simulink model "model_min_mine"  (R2018a)
settings: Solver=ode45  StartTime=0.0  StopTime=20  RelTol=1e-3
(part 8 of 10)

== system model_min_mine/5 систем підйому/4/6-періодні/6-ти періодна пр/постійні ==
  Sum1 : Sum  Inputs=|++++++  SaturateOnIntegerOverflow=on
  Sum2 : Sum  Inputs=|+++  SaturateOnIntegerOverflow=on
  Sum3 : Sum  Inputs=|+++  SaturateOnIntegerOverflow=on
  a1 : Constant  Value=0.5
  a2 : Constant  Value=1.5
  "a4 " : Constant  Value=-1.5
  a5 : Constant  Value=-0.5
  t1 : Constant  Value=0.5
  t2 : Constant  Value=3.5
  t3 : Constant  Value=4
  t4 : Constant  Value=3.5
  "t4/ " : Constant  Value=0.5
  t5 : Constant  Value=0.5
  Out1 : Outport
  Out2 : Outport  Port=2
  Out3 : Outport  Port=3
  Out4 : Outport  Port=4
  Out5 : Outport  Port=5
  Out6 : Outport  Port=6
  Out7 : Outport  Port=7
  Out8 : Outport  Port=8
  Out9 : Outport  Port=9
  Out10 : Outport  Port=10
  wires:
  a1/1 -> Out1/1
  "a4 "/1 -> Out3/1
  a5/1 -> Out4/1
  a2/1 -> Out2/1
  t1/1 -> Out5/1, Sum1/1, Sum2/1
  t3/1 -> Sum1/3, Sum2/3
  t2/1 -> Out6/1, Sum1/2, Sum2/2
  t5/1 -> Sum1/5
  t4/1 -> Out7/1, Sum1/4, Sum3/1
  Sum1/1 -> Out9/1
  Sum2/1 -> Out10/1, Sum3/2
  Sum3/1 -> Out8/1
  "t4/ "/1 -> Sum3/3, Sum1/6

== system model_min_mine/5 систем підйому/4/7-періодні/7-ми періодна криволінійна/Subsystem ==
  t1 : Inport
  t : Inport  Port=2
  a1 : Inport  Port=3
  Constant5 : Constant
  Scope2 : Scope
  Sum4 : Sum  Inputs=|+-  SaturateOnIntegerOverflow=on
  Switch1 : Switch  Criteria=u2 ~= 0  RndMeth=Zero  SaturateOnIntegerOverflow=on
  Генераці : Subsystem  TreatAsAtomicUnit=on
  Out1 : Outport
  wires:
  Генераці/1(Out1) -> Switch1/2
  Sum4/1 -> Генераці/Trigger
  Constant5/1 -> Генераці/1(In1)
  t/1 -> Sum4/2
  t1/1 -> Sum4/1
  Switch1/1 -> Out1/1, Scope2/1
  a1/1 -> Switch1/3

== system model_min_mine/5 систем підйому/4/7-періодні/7-ми періодна криволінійна/Subsystem3 ==
  t1 : Inport
  t : Inport  Port=2
  a1 : Inport  Port=3
  Constant5 : Constant
  Scope2 : Scope
  Sum4 : Sum  Inputs=|+-  SaturateOnIntegerOverflow=on
  Switch1 : Switch  Criteria=u2 ~= 0  RndMeth=Zero  SaturateOnIntegerOverflow=on
  Генераці : Subsystem  TreatAsAtomicUnit=on
  Out1 : Outport
  wires:
  Генераці/1(Out1) -> Switch1/2
  Sum4/1 -> Генераці/Trigger
  Constant5/1 -> Генераці/1(In1)
  t/1 -> Sum4/2
  t1/1 -> Sum4/1
  Switch1/1 -> Out1/1, Scope2/1
  a1/1 -> Switch1/1

== system model_min_mine/5 систем підйому/4/7-періодні/7-ми періодна криволінійна/Subsystem6 ==
  Сума t : Inport
  t : Inport  Port=2
  a : Inport  Port=3
  Constant5 : Constant
  Sum4 : Sum  Inputs=|+-  SaturateOnIntegerOverflow=on
  Switch1 : Switch  Criteria=u2 ~= 0  RndMeth=Zero  SaturateOnIntegerOverflow=on
  Генераці : Subsystem  TreatAsAtomicUnit=on
  Out1 : Outport
  wires:
  Генераці/1(Out1) -> Switch1/2
  Sum4/1 -> Генераці/Trigger
  Constant5/1 -> Генераці/1(In1)
  t/1 -> Sum4/2
  Сума t/1 -> Sum4/1
  Switch1/1 -> Out1/1
  a/1 -> Switch1/3

== system model_min_mine/5 систем підйому/4/7-періодні/7-ми періодна криволінійна/Допоміжний ==
  t1 : Inport
  t : Inport  Port=2
  a1 : Inport  Port=3
  Constant5 : Constant
  Scope2 : Scope
  Sum4 : Sum  Inputs=|+-  SaturateOnIntegerOverflow=on
  Switch1 : Switch  Criteria=u2 ~= 0  RndMeth=Zero  SaturateOnIntegerOverflow=on
  Генераці : Subsystem  TreatAsAtomicUnit=on
  Out1 : Outport
  wires:
  Генераці/1(Out1) -> Switch1/2
  Sum4/1 -> Генераці/Trigger
  Constant5/1 -> Генераці/1(In1)
  t/1 -> Sum4/2
  t1/1 -> Sum4/1
  Switch1/1 -> Out1/1, Scope2/1
  a1/1 -> Switch1/1

== system model_min_mine/5 систем підйому/4/7-періодні/7-ми періодна криволінійна/Допоміжний1 ==
  t1 : Inport
  t : Inport  Port=2
  a1 : Inport  Port=3
  Constant5 : Constant
  Scope2 : Scope
  Sum4 : Sum  Inputs=|+-  SaturateOnIntegerOverflow=on
  Switch1 : Switch  Criteria=u2 ~= 0  RndMeth=Zero  SaturateOnIntegerOverflow=on
  Генераці : Subsystem  TreatAsAtomicUnit=on
  Out1 : Outport
  wires:
  Генераці/1(Out1) -> Switch1/2
  Sum4/1 -> Генераці/Trigger
  Constant5/1 -> Генераці/1(In1)
  t/1 -> Sum4/2
  t1/1 -> Sum4/1
  Switch1/1 -> Out1/1, Scope2/1
  a1/1 -> Switch1/3

== system model_min_mine/5 систем підйому/4/7-періодні/7-ми періодна криволінійна/пакет1 ==
  ti : Inport
  t : Inport  Port=2
  a : Inport  Port=3
  2 : Constant  Value=2
  Math Function1 : Math  Operator=reciprocal  SaturateOnIntegerOverflow=on
  Math Function2 : Math  Operator=reciprocal  SaturateOnIntegerOverflow=on
  Math Function3 : Math  Operator=square  SaturateOnIntegerOverflow=on
  Product10 : Product  Inputs=3  SaturateOnIntegerOverflow=on  OutDataTypeStr=Inherit: Same as first input
  Product3 : Product  Inputs=4  SaturateOnIntegerOverflow=on  OutDataTypeStr=Inherit: Same as first input
  Product4 : Product  SaturateOnIntegerOverflow=on  OutDataTypeStr=Inherit: Same as first input
  Scope1 : Scope
  Scope3 : Scope
  Sum1 : Sum  Inputs=|-+  SaturateOnIntegerOverflow=on
  Sum3 : Sum  Inputs=|+-  SaturateOnIntegerOverflow=on
  Out1 : Outport
  Out2 : Outport  Port=2
  wires:
  Product3/1 -> Sum3/2
  Product4/1 -> Sum3/1
  2/1 -> Math Function2/1
  Math Function1/1 -> Product10/1, Product3/2
  a/1 -> Product4/2, Product3/3, Product10/3, Sum1/2
  ti/1 -> Math Function1/1
  Sum3/1 -> Out2/1, Scope1/1
  Math Function2/1 -> Product3/1
  t/1 -> Math Function3/1, Product10/2, Product4/1
  Math Function3/1 -> Product3/4
  Sum1/1 -> Out1/1, Scope3/1
  Product10/1 -> Sum1/1

== system model_min_mine/5 систем підйому/4/7-періодні/7-ми періодна криволінійна/пакет2 ==
  ti : Inport
  t : Inport  Port=2
  a : Inport  Port=3
  2 : Constant  Value=2
  Math Function1 : Math  Operator=reciprocal  SaturateOnIntegerOverflow=on
  Math Function2 : Math  Operator=reciprocal  SaturateOnIntegerOverflow=on
  Math Function3 : Math  Operator=square  SaturateOnIntegerOverflow=on
  Product10 : Product  Inputs=3  SaturateOnIntegerOverflow=on  OutDataTypeStr=Inherit: Same as first input
  Product3 : Product  Inputs=4  SaturateOnIntegerOverflow=on  OutDataTypeStr=Inherit: Same as first input
  Out1 : Outport
  Out2 : Outport  Port=2
  wires:
  2/1 -> Math Function2/1
  Product10/1 -> Out1/1
  Math Function1/1 -> Product10/1, Product3/2
  a/1 -> Product10/3, Product3/3
  ti/1 -> Math Function1/1
  Math Function2/1 -> Product3/1
  t/1 -> Math Function3/1, Product10/2
  Math Function3/1 -> Product3/4
  Product3/1 -> Out2/1

== system model_min_mine/5 систем підйому/4/7-періодні/7-ми періодна криволінійна/постійні ==
  Sum1 : Sum  Inputs=|+++++++  SaturateOnIntegerOverflow=on
  Sum2 : Sum  Inputs=|+++  SaturateOnIntegerOverflow=on
  Sum3 : Sum  Inputs=|+++  SaturateOnIntegerOverflow=on
  Sum4 : Sum  Inputs=|++  SaturateOnIntegerOverflow=on
  a1 : Constant  Value=0.5
  a2 : Constant  Value=1.5
  "a4 " : Constant  Value=-1.5
  a5 : Constant  Value=-0.5
  t1 : Constant  Value=0.5
  "t1/ " : Constant  Value=0.5
  t2 : Constant  Value=3.5
  t3 : Constant  Value=4
  t4 : Constant  Value=3.5
  "t4/ " : Constant  Value=0.5
  t5 : Constant  Value=0.5
  Out1 : Outport
  Out2 : Outport  Port=2
  Out3 : Outport  Port=3
  Out4 : Outport  Port=4
  Out5 : Outport  Port=5
  Out6 : Outport  Port=6
  Out7 : Outport  Port=7
  Out8 : Outport  Port=8
  Out9 : Outport  Port=9
  Out10 : Outport  Port=10
  Out11 : Outport  Port=11
  wires:
  a1/1 -> Out1/1
  "a4 "/1 -> Out3/1
  a5/1 -> Out4/1
  a2/1 -> Out2/1
  t1/1 -> Out5/1, Sum1/1, Sum2/1, Sum4/1
  t3/1 -> Sum1/3, Sum2/3
  t2/1 -> Out6/1, Sum1/2, Sum2/2
  t5/1 -> Sum1/5
  t4/1 -> Out7/1, Sum1/4, Sum3/1
  Sum1/1 -> Out9/1
  Sum2/1 -> Out10/1, Sum3/2
  Sum3/1 -> Out8/1
  "t4/ "/1 -> Sum3/3, Sum1/6
  "t1/ "/1 -> Sum1/7, Sum4/2
  Sum4/1 -> Out11/1

== system model_min_mine/5 систем підйому/4/7-періодні/7-ми періодна пр/Subsystem ==
  t1 : Inport
  t : Inport  Port=2
  a1 : Inport  Port=3
  Constant5 : Constant
  Scope2 : Scope
  Sum4 : Sum  Inputs=|+-  SaturateOnIntegerOverflow=on
  Switch1 : Switch  Criteria=u2 ~= 0  RndMeth=Zero  SaturateOnIntegerOverflow=on
  Генераці : Subsystem  TreatAsAtomicUnit=on
  Out1 : Outport
  wires:
  Генераці/1(Out1) -> Switch1/2
  Sum4/1 -> Генераці/Trigger
  Constant5/1 -> Генераці/1(In1)
  t/1 -> Sum4/2
  t1/1 -> Sum4/1
  Switch1/1 -> Out1/1, Scope2/1
  a1/1 -> Switch1/3

== system model_min_mine/5 систем підйому/4/7-періодні/7-ми періодна пр/Subsystem1 ==
  t1 : Inport
  t : Inport  Port=2
  a1 : Inport  Port=3
  Constant5 : Constant
  Scope2 : Scope
  Sum4 : Sum  Inputs=|+-  SaturateOnIntegerOverflow=on
  Switch1 : Switch  Criteria=u2 ~= 0  RndMeth=Zero  SaturateOnIntegerOverflow=on
  Генераці : Subsystem  TreatAsAtomicUnit=on
  Out1 : Outport
  wires:
  Генераці/1(Out1) -> Switch1/2
  Sum4/1 -> Генераці/Trigger
  Constant5/1 -> Генераці/1(In1)
  t/1 -> Sum4/2
  t1/1 -> Sum4/1
  Switch1/1 -> Out1/1, Scope2/1
  a1/1 -> Switch1/3

== system model_min_mine/5 систем підйому/4/7-періодні/7-ми періодна пр/Subsystem2 ==
  t1 : Inport
  t : Inport  Port=2
  a1 : Inport  Port=3
  Constant5 : Constant
  Scope2 : Scope
  Scope8 : Scope
  Sum4 : Sum  Inputs=|+-  SaturateOnIntegerOverflow=on
  Switch1 : Switch  Criteria=u2 ~= 0  RndMeth=Zero  SaturateOnIntegerOverflow=on
  Генераці : Subsystem  TreatAsAtomicUnit=on
  Out1 : Outport
  wires:
  Генераці/1(Out1) -> Switch1/2
  Sum4/1 -> Генераці/Trigger
  Constant5/1 -> Генераці/1(In1)
  t/1 -> Sum4/2
  t1/1 -> Sum4/1
  Switch1/1 -> Scope2/1, Out1/1, Scope8/1
  a1/1 -> Switch1/1

== system model_min_mine/5 систем підйому/4/7-періодні/7-ми періодна пр/Subsystem3 ==
  t1 : Inport
  t : Inport  Port=2
  a1 : Inport  Port=3
  Constant5 : Constant
  Scope2 : Scope
  Sum4 : Sum  Inputs=|+-  SaturateOnIntegerOverflow=on
  Switch1 : Switch  Criteria=u2 ~= 0  RndMeth=Zero  SaturateOnIntegerOverflow=on
  Генераці : Subsystem  TreatAsAtomicUnit=on
  Out1 : Outport
  wires:
  Генераці/1(Out1) -> Switch1/2
  Sum4/1 -> Генераці/Trigger
  Constant5/1 -> Генераці/1(In1)
  t/1 -> Sum4/2
  t1/1 -> Sum4/1
  Switch1/1 -> Out1/1, Scope2/1
  a1/1 -> Switch1/1

== system model_min_mine/5 систем підйому/4/7-періодні/7-ми періодна пр/Subsystem6 ==
  Сума t : Inport
  t : Inport  Port=2
  a : Inport  Port=3
  Constant5 : Constant
  Sum4 : Sum  Inputs=|+-  SaturateOnIntegerOverflow=on
  Switch1 : Switch  Criteria=u2 ~= 0  RndMeth=Zero  SaturateOnIntegerOverflow=on
  Генераці : Subsystem  TreatAsAtomicUnit=on
  Out1 : Outport
  wires:
  Генераці/1(Out1) -> Switch1/2
  Sum4/1 -> Генераці/Trigger
  Constant5/1 -> Генераці/1(In1)
  t/1 -> Sum4/2
  Сума t/1 -> Sum4/1
  Switch1/1 -> Out1/1
  a/1 -> Switch1/3

== system model_min_mine/5 систем підйому/4/7-періодні/7-ми періодна пр/Допоміжний ==
  t1 : Inport
  t : Inport  Port=2
  a1 : Inport  Port=3
  Constant5 : Constant
  Scope2 : Scope
  Sum4 : Sum  Inputs=|+-  SaturateOnIntegerOverflow=on
  Switch1 : Switch  Criteria=u2 ~= 0  RndMeth=Zero  SaturateOnIntegerOverflow=on
  Генераці : Subsystem  TreatAsAtomicUnit=on
  Out1 : Outport
  wires:
  Генераці/1(Out1) -> Switch1/2
  Sum4/1 -> Генераці/Trigger
  Constant5/1 -> Генераці/1(In1)
  t/1 -> Sum4/2
  t1/1 -> Sum4/1
  Switch1/1 -> Out1/1, Scope2/1
  a1/1 -> Switch1/1

== system model_min_mine/5 систем підйому/4/7-періодні/7-ми періодна пр/Допоміжний1 ==
  t1 : Inport
  t : Inport  Port=2
  a1 : Inport  Port=3
  Constant5 : Constant
  Scope2 : Scope
  Sum4 : Sum  Inputs=|+-  SaturateOnIntegerOverflow=on
  Switch1 : Switch  Criteria=u2 ~= 0  RndMeth=Zero  SaturateOnIntegerOverflow=on
  Генераці : Subsystem  TreatAsAtomicUnit=on
  Out1 : Outport
  wires:
  Генераці/1(Out1) -> Switch1/2
  Sum4/1 -> Генераці/Trigger
  Constant5/1 -> Генераці/1(In1)
  t/1 -> Sum4/2
  t1/1 -> Sum4/1
  Switch1/1 -> Out1/1, Scope2/1
  a1/1 -> Switch1/3

== system model_min_mine/5 систем підйому/4/7-періодні/7-ми періодна пр/постійні ==
  Sum1 : Sum  Inputs=|+++++++  SaturateOnIntegerOverflow=on
  Sum2 : Sum  Inputs=|+++  SaturateOnIntegerOverflow=on
  Sum3 : Sum  Inputs=|+++  SaturateOnIntegerOverflow=on
  Sum4 : Sum  Inputs=|++  SaturateOnIntegerOverflow=on
  a1 : Constant  Value=0.5
  a2 : Constant  Value=1.5
  "a4 " : Constant  Value=-1.5
  a5 : Constant  Value=-0.5
  t1 : Constant  Value=0.5
  "t1/ " : Constant  Value=0.5
  t2 : Constant  Value=3.5
  t3 : Constant  Value=8
  t4 : Constant  Value=3.5
  "t4/ " : Constant  Value=0.5
  t5 : Constant  Value=0.5
  Out1 : Outport
  Out2 : Outport  Port=2
  Out3 : Outport  Port=3
  Out4 : Outport  Port=4
  Out5 : Outport  Port=5
  Out6 : Outport  Port=6
  Out7 : Outport  Port=7
  Out8 : Outport  Port=8
  Out9 : Outport  Port=9
  Out10 : Outport  Port=10
  Out11 : Outport  Port=11
  wires:
  a1/1 -> Out1/1
  "a4 "/1 -> Out3/1
  a5/1 -> Out4/1
  a2/1 -> Out2/1
  t1/1 -> Out5/1, Sum1/1, Sum2/1, Sum4/1
  t3/1 -> Sum1/3, Sum2/3
  t2/1 -> Out6/1, Sum1/2, Sum2/2
  t5/1 -> Sum1/5
  t4/1 -> Out7/1, Sum1/4, Sum3/1
  Sum1/1 -> Out9/1
  Sum2/1 -> Out10/1, Sum3/2
  Sum3/1 -> Out8/1
  "t4/ "/1 -> Sum3/3, Sum1/6
  "t1/ "/1 -> Sum1/7, Sum4/2
  Sum4/1 -> Out11/1

== system model_min_mine/5 систем підйому/6/3-періодні/Криволінійна-3/Генераці1 ==
  In1 : Inport
  Trigger : TriggerPort  TriggerType=either  VariantControl=(inherit)  ShowOutputPort=on
  Out1 : Outport
  wires:
  In1/1 -> Out1/1

== system model_min_mine/5 систем підйому/6/3-періодні/Криволінійна-3/пакет2 ==
  ti : Inport
  t : Inport  Port=2
  a : Inport  Port=3
  2 : Constant  Value=2
  Math Function1 : Math  Operator=reciprocal  SaturateOnIntegerOverflow=on
  Math Function2 : Math  Operator=reciprocal  SaturateOnIntegerOverflow=on
  Math Function3 : Math  Operator=square  SaturateOnIntegerOverflow=on
  Product10 : Product  Inputs=3  SaturateOnIntegerOverflow=on  OutDataTypeStr=Inherit: Same as first input
  Product3 : Product  Inputs=4  SaturateOnIntegerOverflow=on  OutDataTypeStr=Inherit: Same as first input
  Product4 : Product  SaturateOnIntegerOverflow=on  OutDataTypeStr=Inherit: Same as first input
  Scope1 : Scope
  Scope3 : Scope
  Sum1 : Sum  Inputs=|-+  SaturateOnIntegerOverflow=on
  Sum3 : Sum  Inputs=|+-  SaturateOnIntegerOverflow=on
  Out1 : Outport
  Out2 : Outport  Port=2
  wires:
  Product3/1 -> Sum3/2
  Product4/1 -> Sum3/1
  2/1 -> Math Function2/1
  Math Function1/1 -> Product10/1, Product3/2
  a/1 -> Product4/2, Product3/3, Product10/3, Sum1/2
  ti/1 -> Math Function1/1
  Sum3/1 -> Out2/1, Scope1/1
  Math Function2/1 -> Product3/1
  t/1 -> Math Function3/1, Product10/2, Product4/1
  Math Function3/1 -> Product3/4
  Sum1/1 -> Out1/1, Scope3/1
  Product10/1 -> Sum1/1

== system model_min_mine/5 систем підйому/6/3-періодні/Криволінійна-3/пакет3 ==
  ti : Inport
  t : Inport  Port=2
  a : Inport  Port=3
  2 : Constant  Value=2
  Math Function1 : Math  Operator=reciprocal  SaturateOnIntegerOverflow=on
  Math Function2 : Math  Operator=reciprocal  SaturateOnIntegerOverflow=on
  Math Function3 : Math  Operator=square  SaturateOnIntegerOverflow=on
  Product10 : Product  Inputs=3  SaturateOnIntegerOverflow=on  OutDataTypeStr=Inherit: Same as first input
  Product3 : Product  Inputs=4  SaturateOnIntegerOverflow=on  OutDataTypeStr=Inherit: Same as first input
  Out1 : Outport
  Out2 : Outport  Port=2
  wires:
  2/1 -> Math Function2/1
  Product10/1 -> Out1/1
  Math Function1/1 -> Product10/1, Product3/2
  a/1 -> Product10/3, Product3/3
  ti/1 -> Math Function1/1
  Math Function2/1 -> Product3/1
  t/1 -> Math Function3/1, Product10/2
  Math Function3/1 -> Product3/4
  Product3/1 -> Out2/1

== system model_min_mine/5 систем підйому/6/3-періодні/Криволінійна-3/постійні ==
  a1 : Constant  Value=0.3
  a3 : Constant  Value=-0.3
  t1 : Constant  Value=1.15
  t3 : Constant  Value=1.15
  Out1 : Outport
  Out2 : Outport  Port=2
  Out3 : Outport  Port=3
  Out4 : Outport  Port=4
  wires:
  a1/1 -> Out1/1
  t1/1 -> Out3/1
  a3/1 -> Out2/1
  t3/1 -> Out4/1

== system model_min_mine/5 систем підйому/6/3-періодні/Пр/Генераці ==
  In1 : Inport
  Trigger : TriggerPort  TriggerType=either  VariantControl=(inherit)  ShowOutputPort=on
  Out1 : Outport
  wires:
  In1/1 -> Out1/1

== system model_min_mine/5 систем підйому/6/3-періодні/Пр/Генераці1 ==
  In1 : Inport
  Trigger : TriggerPort  TriggerType=either  VariantControl=(inherit)  ShowOutputPort=on
  Out1 : Outport
  wires:
  In1/1 -> Out1/1

== system model_min_mine/5 систем підйому/6/3-періодні/Пр/Генераці2 ==
  In1 : Inport
  Trigger : TriggerPort  TriggerType=either  VariantControl=(inherit)  ShowOutputPort=on
  Out1 : Outport
  wires:
  In1/1 -> Out1/1

== system model_min_mine/5 систем підйому/6/3-періодні/Пр/постійні ==
  (t1) : Constant  Value=1.15
  (t2) : Constant  Value=2
  (t3) : Constant  Value=1.15
  Sum1 : Sum  Inputs=|++  SaturateOnIntegerOverflow=on
  a1 : Constant  Value=0.3
  a3 : Constant  Value=-0.3
  Out1 : Outport
  Out2 : Outport  Port=2
  Out3 : Outport  Port=3
  Out4 : Outport  Port=4
  Out5 : Outport  Port=5
  wires:
  a1/1 -> Out1/1
  a3/1 -> Out2/1
  (t3)/1 -> Out3/1
  (t1)/1 -> Out4/1, Sum1/1
  (t2)/1 -> Sum1/2
  Sum1/1 -> Out5/1

== system model_min_mine/5 систем підйому/6/5-періодні/криво/Subsystem ==
  t1 : Inport
  t : Inport  Port=2
  a1 : Inport  Port=3
  Constant5 : Constant
  Scope2 : Scope
  Sum4 : Sum  Inputs=|+-  SaturateOnIntegerOverflow=on
  Switch1 : Switch  Criteria=u2 ~= 0  RndMeth=Zero  SaturateOnIntegerOverflow=on
  Генераці : Subsystem  TreatAsAtomicUnit=on
  Out1 : Outport
  wires:
  Генераці/1(Out1) -> Switch1/2
  Sum4/1 -> Генераці/Trigger
  Constant5/1 -> Генераці/1(In1)
  t/1 -> Sum4/2
  t1/1 -> Sum4/1
  Switch1/1 -> Out1/1, Scope2/1
  a1/1 -> Switch1/3

== system model_min_mine/5 систем підйому/6/5-періодні/криво/Subsystem1 ==
  t1 : Inport
  t : Inport  Port=2
  a1 : Inport  Port=3
  Constant5 : Constant
  Scope2 : Scope
  Sum4 : Sum  Inputs=|+-  SaturateOnIntegerOverflow=on
  Switch1 : Switch  Criteria=u2 ~= 0  RndMeth=Zero  SaturateOnIntegerOverflow=on
  Генераці : Subsystem  TreatAsAtomicUnit=on
  Out1 : Outport
  wires:
  Генераці/1(Out1) -> Switch1/2
  Sum4/1 -> Генераці/Trigger
  Constant5/1 -> Генераці/1(In1)
  t/1 -> Sum4/2
  t1/1 -> Sum4/1
  Switch1/1 -> Out1/1, Scope2/1
  a1/1 -> Switch1/3

== system model_min_mine/5 систем підйому/6/5-періодні/криво/Subsystem2 ==
  t1 : Inport
  t : Inport  Port=2
  a1 : Inport  Port=3
  Constant5 : Constant
  Scope2 : Scope
  Scope8 : Scope
  Sum4 : Sum  Inputs=|+-  SaturateOnIntegerOverflow=on
  Switch1 : Switch  Criteria=u2 ~= 0  RndMeth=Zero  SaturateOnIntegerOverflow=on
  Генераці : Subsystem  TreatAsAtomicUnit=on
  Out1 : Outport
  wires:
  Генераці/1(Out1) -> Switch1/2
  Sum4/1 -> Генераці/Trigger
  Constant5/1 -> Генераці/1(In1)
  t/1 -> Sum4/2
  t1/1 -> Sum4/1
  Switch1/1 -> Scope2/1, Out1/1, Scope8/1
  a1/1 -> Switch1/1

== system model_min_mine/5 систем підйому/6/5-періодні/криво/Subsystem3 ==
  t1 : Inport
  t : Inport  Port=2
  a1 : Inport  Port=3
  Constant5 : Constant
  Scope2 : Scope
  Sum4 : Sum  Inputs=|+-  SaturateOnIntegerOverflow=on
  Switch1 : Switch  Criteria=u2 ~= 0  RndMeth=Zero  SaturateOnIntegerOverflow=on
  Генераці : Subsystem  TreatAsAtomicUnit=on
  Out1 : Outport
  wires:
  Генераці/1(Out1) -> Switch1/2
  Sum4/1 -> Генераці/Trigger
  Constant5/1 -> Генераці/1(In1)
  t/1 -> Sum4/2
  t1/1 -> Sum4/1
  Switch1/1 -> Out1/1, Scope2/1
  a1/1 -> Switch1/1

== system model_min_mine/5 систем підйому/6/5-періодні/криво/Subsystem6 ==
  Сума t : Inport
  t : Inport  Port=2
  a : Inport  Port=3
  Constant5 : Constant
  Sum4 : Sum  Inputs=|+-  SaturateOnIntegerOverflow=on
  Switch1 : Switch  Criteria=u2 ~= 0  RndMeth=Zero  SaturateOnIntegerOverflow=on
  Генераці : Subsystem  TreatAsAtomicUnit=on
  Out1 : Outport
  wires:
  Генераці/1(Out1) -> Switch1/2
  Sum4/1 -> Генераці/Trigger
  Constant5/1 -> Генераці/1(In1)
  t/1 -> Sum4/2
  Сума t/1 -> Sum4/1
  Switch1/1 -> Out1/1
  a/1 -> Switch1/3

== system model_min_mine/5 систем підйому/6/5-періодні/криво/Допоміжний ==
  t1 : Inport
  t : Inport  Port=2
  a1 : Inport  Port=3
  Constant5 : Constant
  Scope2 : Scope
  Sum4 : Sum  Inputs=|+-  SaturateOnIntegerOverflow=on
  Switch1 : Switch  Criteria=u2 ~= 0  RndMeth=Zero  SaturateOnIntegerOverflow=on
  Генераці : Subsystem  TreatAsAtomicUnit=on
  Out1 : Outport
  wires:
  Генераці/1(Out1) -> Switch1/2
  Sum4/1 -> Генераці/Trigger
  Constant5/1 -> Генераці/1(In1)
  t/1 -> Sum4/2
  t1/1 -> Sum4/1
  Switch1/1 -> Out1/1, Scope2/1
  a1/1 -> Switch1/1

== system model_min_mine/5 систем підйому/6/5-періодні/криво/Допоміжний1 ==
  t1 : Inport
  t : Inport  Port=2
  a1 : Inport  Port=3
  Constant5 : Constant
  Scope2 : Scope
  Sum4 : Sum  Inputs=|+-  SaturateOnIntegerOverflow=on
  Switch1 : Switch  Criteria=u2 ~= 0  RndMeth=Zero  SaturateOnIntegerOverflow=on
  Генераці : Subsystem  TreatAsAtomicUnit=on
  Out1 : Outport
  wires:
  Генераці/1(Out1) -> Switch1/2
  Sum4/1 -> Генераці/Trigger
  Constant5/1 -> Генераці/1(In1)
  t/1 -> Sum4/2
  t1/1 -> Sum4/1
  Switch1/1 -> Out1/1, Scope2/1
  a1/1 -> Switch1/3

== system model_min_mine/5 систем підйому/6/5-періодні/криво/постійні ==
  Sum1 : Sum  Inputs=|+++++  SaturateOnIntegerOverflow=on
  Sum2 : Sum  Inputs=|+++  SaturateOnIntegerOverflow=on
  Sum3 : Sum  Inputs=|++  SaturateOnIntegerOverflow=on
  a1 : Constant  Value=0.5
  a2 : Constant  Value=1.5
  "a4 " : Constant  Value=-1.5
  a5 : Constant  Value=-0.5
  t1 : Constant  Value=0.5
  t2 : Constant  Value=3.5
  t3 : Constant  Value=4
  t4 : Constant  Value=3.5
  t5 : Constant  Value=0.5
  Out1 : Outport
  Out2 : Outport  Port=2
  Out3 : Outport  Port=3
  Out4 : Outport  Port=4
  Out5 : Outport  Port=5
  Out6 : Outport  Port=6
  Out7 : Outport  Port=7
  Out8 : Outport  Port=8
  Out9 : Outport  Port=9
  Out10 : Outport  Port=10
  wires:
  a1/1 -> Out1/1
  "a4 "/1 -> Out3/1
  a5/1 -> Out4/1
  a2/1 -> Out2/1
  t1/1 -> Out5/1, Sum1/1, Sum2/1
  t3/1 -> Sum1/3, Sum2/3
  t2/1 -> Out6/1, Sum1/2, Sum2/2
  t5/1 -> Sum1/5
  t4/1 -> Out7/1, Sum1/4, Sum3/1
  Sum1/1 -> Out9/1
  Sum2/1 -> Out10/1, Sum3/2
  Sum3/1 -> Out8/1

== system model_min_mine/5 систем підйому/6/5-періодні/пр/Subsystem ==
  t1 : Inport
  t : Inport  Port=2
  a1 : Inport  Port=3
  Constant5 : Constant
  Scope2 : Scope
  Sum4 : Sum  Inputs=|+-  SaturateOnIntegerOverflow=on
  Switch1 : Switch  Criteria=u2 ~= 0  RndMeth=Zero  SaturateOnIntegerOverflow=on
  Генераці : Subsystem  TreatAsAtomicUnit=on
  Out1 : Outport
  wires:
  Генераці/1(Out1) -> Switch1/2
  Sum4/1 -> Генераці/Trigger
  Constant5/1 -> Генераці/1(In1)
  t/1 -> Sum4/2
  t1/1 -> Sum4/1
  Switch1/1 -> Out1/1, Scope2/1
  a1/1 -> Switch1/3

== system model_min_mine/5 систем підйому/6/5-періодні/пр/Subsystem1 ==
  t1 : Inport
  t : Inport  Port=2
  a1 : Inport  Port=3
  Constant5 : Constant
  Scope2 : Scope
  Sum4 : Sum  Inputs=|+-  SaturateOnIntegerOverflow=on
  Switch1 : Switch  Criteria=u2 ~= 0  RndMeth=Zero  SaturateOnIntegerOverflow=on
  Генераці : Subsystem  TreatAsAtomicUnit=on
  Out1 : Outport
  wires:
  Генераці/1(Out1) -> Switch1/2
  Sum4/1 -> Генераці/Trigger
  Constant5/1 -> Генераці/1(In1)
  t/1 -> Sum4/2
  t1/1 -> Sum4/1
  Switch1/1 -> Out1/1, Scope2/1
  a1/1 -> Switch1/3

== system model_min_mine/5 систем підйому/6/5-періодні/пр/Subsystem4 ==
  ti : Inport
  t : Inport  Port=2
  a : Inport  Port=3
  Constant5 : Constant
  Sum4 : Sum  Inputs=|+-  SaturateOnIntegerOverflow=on
  Switch1 : Switch  Criteria=u2 ~= 0  RndMeth=Zero  SaturateOnIntegerOverflow=on
  Генераці : Subsystem  TreatAsAtomicUnit=on
  Out1 : Outport
  wires:
  Генераці/1(Out1) -> Switch1/2
  Sum4/1 -> Генераці/Trigger
  Constant5/1 -> Генераці/1(In1)
  t/1 -> Sum4/2
  ti/1 -> Sum4/1
  a/1 -> Switch1/1
  Switch1/1 -> Out1/1

== system model_min_mine/5 систем підйому/6/5-періодні/пр/Subsystem5 ==
  ti : Inport
  t : Inport  Port=2
  a : Inport  Port=3
  Constant5 : Constant
  Sum4 : Sum  Inputs=|+-  SaturateOnIntegerOverflow=on
  Switch1 : Switch  Criteria=u2 ~= 0  RndMeth=Zero  SaturateOnIntegerOverflow=on
  Генераці : Subsystem  TreatAsAtomicUnit=on
  Out1 : Outport
  wires:
  Генераці/1(Out1) -> Switch1/2
  Sum4/1 -> Генераці/Trigger
  Constant5/1 -> Генераці/1(In1)
  t/1 -> Sum4/2
  ti/1 -> Sum4/1
  a/1 -> Switch1/1
  Switch1/1 -> Out1/1

== system model_min_mine/5 систем підйому/6/5-періодні/пр/Subsystem6 ==
  Сума t : Inport
  t : Inport  Port=2
  a : Inport  Port=3
  Constant5 : Constant
  Sum4 : Sum  Inputs=|+-  SaturateOnIntegerOverflow=on
  Switch1 : Switch  Criteria=u2 ~= 0  RndMeth=Zero  SaturateOnIntegerOverflow=on
  Генераці : Subsystem  TreatAsAtomicUnit=on
  Out1 : Outport
  wires:
  Генераці/1(Out1) -> Switch1/2
  Sum4/1 -> Генераці/Trigger
  Constant5/1 -> Генераці/1(In1)
  t/1 -> Sum4/2
  Сума t/1 -> Sum4/1
  Switch1/1 -> Out1/1
  a/1 -> Switch1/3

== system model_min_mine/5 систем підйому/6/5-періодні/пр/Допоміжний ==
  t1 : Inport
  t : Inport  Port=2
  a1 : Inport  Port=3
  Constant5 : Constant
  Scope2 : Scope
  Sum4 : Sum  Inputs=|+-  SaturateOnIntegerOverflow=on
  Switch1 : Switch  Criteria=u2 ~= 0  RndMeth=Zero  SaturateOnIntegerOverflow=on
  Генераці : Subsystem  TreatAsAtomicUnit=on
  Out1 : Outport
  wires:
  Генераці/1(Out1) -> Switch1/2
  Sum4/1 -> Генераці/Trigger
  Constant5/1 -> Генераці/1(In1)
  t/1 -> Sum4/2
  t1/1 -> Sum4/1
  Switch1/1 -> Out1/1, Scope2/1
  a1/1 -> Switch1/1

== system model_min_mine/5 систем підйому/6/5-періодні/пр/Допоміжний -1 ==
  t1 : Inport
  t : Inport  Port=2
  a1 : Inport  Port=3
  Constant5 : Constant
  Scope2 : Scope
  Sum4 : Sum  Inputs=|+-  SaturateOnIntegerOverflow=on
  Switch1 : Switch  Criteria=u2 ~= 0  RndMeth=Zero  SaturateOnIntegerOverflow=on
  Генераці : Subsystem  TreatAsAtomicUnit=on
  Out1 : Outport
  wires:
  Генераці/1(Out1) -> Switch1/2
  Sum4/1 -> Генераці/Trigger
  Constant5/1 -> Генераці/1(In1)
  t/1 -> Sum4/2
  t1/1 -> Sum4/1
  Switch1/1 -> Out1/1, Scope2/1
  a1/1 -> Switch1/1

== system model_min_mine/5 систем підйому/6/5-періодні/пр/Допоміжний -2 ==
  t1 : Inport
  t : Inport  Port=2
  a1 : Inport  Port=3
  Constant5 : Constant
  Scope2 : Scope
  Sum4 : Sum  Inputs=|+-  SaturateOnIntegerOverflow=on
  Switch1 : Switch  Criteria=u2 ~= 0  RndMeth=Zero  SaturateOnIntegerOverflow=on
  Генераці : Subsystem  TreatAsAtomicUnit=on
  Out1 : Outport
  wires:
  Генераці/1(Out1) -> Switch1/2
  Sum4/1 -> Генераці/Trigger
  Constant5/1 -> Генераці/1(In1)
  t/1 -> Sum4/2
  t1/1 -> Sum4/1
  Switch1/1 -> Out1/1, Scope2/1
  a1/1 -> Switch1/1

== system model_min_mine/5 систем підйому/6/5-періодні/пр/Допоміжний -3 ==
  t1 : Inport
  t : Inport  Port=2
  a1 : Inport  Port=3
  Constant5 : Constant
  Scope2 : Scope
  Sum4 : Sum  Inputs=|+-  SaturateOnIntegerOverflow=on
  Switch1 : Switch  Criteria=u2 ~= 0  RndMeth=Zero  SaturateOnIntegerOverflow=on
  Генераці : Subsystem  TreatAsAtomicUnit=on
  Out1 : Outport
  wires:
  Генераці/1(Out1) -> Switch1/2
  Sum4/1 -> Генераці/Trigger
  Constant5/1 -> Генераці/1(In1)
  t/1 -> Sum4/2
  t1/1 -> Sum4/1
  Switch1/1 -> Out1/1, Scope2/1
  a1/1 -> Switch1/1

== system model_min_mine/5 систем підйому/6/5-періодні/пр/Допоміжний -4 ==
  t1 : Inport
  t : Inport  Port=2
  a1 : Inport  Port=3
  Constant5 : Constant
  Scope2 : Scope
  Sum4 : Sum  Inputs=|+-  SaturateOnIntegerOverflow=on
  Switch1 : Switch  Criteria=u2 ~= 0  RndMeth=Zero  SaturateOnIntegerOverflow=on
  Генераці : Subsystem  TreatAsAtomicUnit=on
  Out1 : Outport
  wires:
  Генераці/1(Out1) -> Switch1/2
  Sum4/1 -> Генераці/Trigger
  Constant5/1 -> Генераці/1(In1)
  t/1 -> Sum4/2
  t1/1 -> Sum4/1
  Switch1/1 -> Out1/1, Scope2/1
  a1/1 -> Switch1/1

== system model_min_mine/5 систем підйому/6/5-періодні/пр/пакет1 ==
  ti : Inport
  t : Inport  Port=2
  a : Inport  Port=3
  2 : Constant  Value=2
  Math Function1 : Math  Operator=reciprocal  SaturateOnIntegerOverflow=on
  Math Function2 : Math  Operator=reciprocal  SaturateOnIntegerOverflow=on
  Math Function3 : Math  Operator=square  SaturateOnIntegerOverflow=on
  Product10 : Product  Inputs=3  SaturateOnIntegerOverflow=on  OutDataTypeStr=Inherit: Same as first input
  Product3 : Product  Inputs=4  SaturateOnIntegerOverflow=on  OutDataTypeStr=Inherit: Same as first input
  Product4 : Product  SaturateOnIntegerOverflow=on  OutDataTypeStr=Inherit: Same as first input
  Scope3 : Scope
  Sum1 : Sum  Inputs=|-+  SaturateOnIntegerOverflow=on
  Sum3 : Sum  Inputs=|+-  SaturateOnIntegerOverflow=on
  Out1 : Outport
  Out2 : Outport  Port=2
  wires:
  Product3/1 -> Sum3/2
  Product4/1 -> Sum3/1
  2/1 -> Math Function2/1
  Math Function1/1 -> Product10/1, Product3/2
  a/1 -> Product4/2, Product3/3, Product10/3, Sum1/2
  ti/1 -> Math Function1/1
  Sum3/1 -> Out2/1
  Math Function2/1 -> Product3/1
  t/1 -> Math Function3/1, Product10/2, Product4/1
  Math Function3/1 -> Product3/4
  Sum1/1 -> Out1/1, Scope3/1
  Product10/1 -> Sum1/1

== system model_min_mine/5 систем підйому/6/5-періодні/пр/пакет2 ==
  ti : Inport
  t : Inport  Port=2
  a : Inport  Port=3
  2 : Constant  Value=2
  Math Function1 : Math  Operator=reciprocal  SaturateOnIntegerOverflow=on
  Math Function2 : Math  Operator=reciprocal  SaturateOnIntegerOverflow=on
  Math Function3 : Math  Operator=square  SaturateOnIntegerOverflow=on
  Product10 : Product  Inputs=3  SaturateOnIntegerOverflow=on  OutDataTypeStr=Inherit: Same as first input
  Product3 : Product  Inputs=4  SaturateOnIntegerOverflow=on  OutDataTypeStr=Inherit: Same as first input
  Out1 : Outport
  Out2 : Outport  Port=2
  wires:
  2/1 -> Math Function2/1
  Product10/1 -> Out1/1
  Math Function1/1 -> Product10/1, Product3/2
  a/1 -> Product10/3, Product3/3
  ti/1 -> Math Function1/1
  Math Function2/1 -> Product3/1
  t/1 -> Math Function3/1, Product10/2
  Math Function3/1 -> Product3/4
  Product3/1 -> Out2/1

== system model_min_mine/5 систем підйому/6/5-періодні/пр/постійні ==
  Sum1 : Sum  Inputs=|+++++++  SaturateOnIntegerOverflow=on
  a1 : Constant  Value=0.5
  a2 : Constant  Value=1.5
  "a3 " : Constant  Value=1.5
  a5 на кінці : Constant  Value=-1.5
  a6 : Constant  Value=-1.5
  a7 : Constant  Value=-0.5
  t{1,3,5,7} (4 alike) : Constant  Value=0.5
  t2 : Constant  Value=3.5
  t4 : Constant  Value=3
  t6 : Constant  Value=3.5
  Out1 : Outport
  Out2 : Outport  Port=2
  Out3 : Outport  Port=3
  Out4 : Outport  Port=4
  Out5 : Outport  Port=5
  Out6 : Outport  Port=6
  Out7 : Outport  Port=7
  Out8 : Outport  Port=8
  Out9 : Outport  Port=9
  Out10 : Outport  Port=10
  Out11 : Outport  Port=11
  Out12 : Outport  Port=12
  Out13 : Outport  Port=13
  wires:
  a1/1 -> Out1/1
  "a3 "/1 -> Out3/1
  a5 на кінці/1 -> Out4/1
  a2/1 -> Out2/1
  a6/1 -> Out5/1
  a7/1 -> Out6/1
  t1/1 -> Out7/1, Sum1/1
  t3/1 -> Out9/1, Sum1/3
  t2/1 -> Out8/1, Sum1/2
  t5/1 -> Out11/1, Sum1/5
  t6/1 -> Out12/1, Sum1/6
  t7/1 -> Out13/1, Sum1/7
  t4/1 -> Sum1/4
  Sum1/1 -> Out10/1

== system model_min_mine/5 систем підйому/6/6-періодні/6-ти періодна криволінійна/Subsystem ==
  t1 : Inport
  t : Inport  Port=2
  a1 : Inport  Port=3
  Constant5 : Constant
  Scope2 : Scope
  Sum4 : Sum  Inputs=|+-  SaturateOnIntegerOverflow=on
  Switch1 : Switch  Criteria=u2 ~= 0  RndMeth=Zero  SaturateOnIntegerOverflow=on
  Генераці : Subsystem  TreatAsAtomicUnit=on
  Out1 : Outport
  wires:
  Генераці/1(Out1) -> Switch1/2
  Sum4/1 -> Генераці/Trigger
  Constant5/1 -> Генераці/1(In1)
  t/1 -> Sum4/2
  t1/1 -> Sum4/1
  Switch1/1 -> Out1/1, Scope2/1
  a1/1 -> Switch1/3

== system model_min_mine/5 систем підйому/6/6-періодні/6-ти періодна криволінійна/Subsystem3 ==
  t1 : Inport
  t : Inport  Port=2
  a1 : Inport  Port=3
  Constant5 : Constant
  Scope2 : Scope
  Sum4 : Sum  Inputs=|+-  SaturateOnIntegerOverflow=on
  Switch1 : Switch  Criteria=u2 ~= 0  RndMeth=Zero  SaturateOnIntegerOverflow=on
  Генераці : Subsystem  TreatAsAtomicUnit=on
  Out1 : Outport
  wires:
  Генераці/1(Out1) -> Switch1/2
  Sum4/1 -> Генераці/Trigger
  Constant5/1 -> Генераці/1(In1)
  t/1 -> Sum4/2
  t1/1 -> Sum4/1
  Switch1/1 -> Out1/1, Scope2/1
  a1/1 -> Switch1/1

== system model_min_mine/5 систем підйому/6/6-періодні/6-ти періодна криволінійна/Subsystem6 ==
  Сума t : Inport
  t : Inport  Port=2
  a : Inport  Port=3
  Constant5 : Constant
  Sum4 : Sum  Inputs=|+-  SaturateOnIntegerOverflow=on
  Switch1 : Switch  Criteria=u2 ~= 0  RndMeth=Zero  SaturateOnIntegerOverflow=on
  Генераці : Subsystem  TreatAsAtomicUnit=on
  Out1 : Outport
  wires:
  Генераці/1(Out1) -> Switch1/2
  Sum4/1 -> Генераці/Trigger
  Constant5/1 -> Генераці/1(In1)
  t/1 -> Sum4/2
  Сума t/1 -> Sum4/1
  Switch1/1 -> Out1/1
  a/1 -> Switch1/3

== system model_min_mine/5 систем підйому/6/6-періодні/6-ти періодна криволінійна/Допоміжний ==
  t1 : Inport
  t : Inport  Port=2
  a1 : Inport  Port=3
  Constant5 : Constant
  Scope2 : Scope
  Sum4 : Sum  Inputs=|+-  SaturateOnIntegerOverflow=on
  Switch1 : Switch  Criteria=u2 ~= 0  RndMeth=Zero  SaturateOnIntegerOverflow=on
  Генераці : Subsystem  TreatAsAtomicUnit=on
  Out1 : Outport
  wires:
  Генераці/1(Out1) -> Switch1/2
  Sum4/1 -> Генераці/Trigger
  Constant5/1 -> Генераці/1(In1)
  t/1 -> Sum4/2
  t1/1 -> Sum4/1
  Switch1/1 -> Out1/1, Scope2/1
  a1/1 -> Switch1/1

== system model_min_mine/5 систем підйому/6/6-періодні/6-ти періодна криволінійна/Допоміжний1 ==
  t1 : Inport
  t : Inport  Port=2
  a1 : Inport  Port=3
  Constant5 : Constant
  Scope2 : Scope
  Sum4 : Sum  Inputs=|+-  SaturateOnIntegerOverflow=on
  Switch1 : Switch  Criteria=u2 ~= 0  RndMeth=Zero  SaturateOnIntegerOverflow=on
  Генераці : Subsystem  TreatAsAtomicUnit=on
  Out1 : Outport
  wires:
  Генераці/1(Out1) -> Switch1/2
  Sum4/1 -> Генераці/Trigger
  Constant5/1 -> Генераці/1(In1)
  t/1 -> Sum4/2
  t1/1 -> Sum4/1
  Switch1/1 -> Out1/1, Scope2/1
  a1/1 -> Switch1/3

== system model_min_mine/5 систем підйому/6/6-періодні/6-ти періодна криволінійна/пакет1 ==
  ti : Inport
  t : Inport  Port=2
  a : Inport  Port=3
  2 : Constant  Value=2
  Math Function1 : Math  Operator=reciprocal  SaturateOnIntegerOverflow=on
  Math Function2 : Math  Operator=reciprocal  SaturateOnIntegerOverflow=on
  Math Function3 : Math  Operator=square  SaturateOnIntegerOverflow=on
  Product10 : Product  Inputs=3  SaturateOnIntegerOverflow=on  OutDataTypeStr=Inherit: Same as first input
  Product3 : Product  Inputs=4  SaturateOnIntegerOverflow=on  OutDataTypeStr=Inherit: Same as first input
  Product4 : Product  SaturateOnIntegerOverflow=on  OutDataTypeStr=Inherit: Same as first input
  Scope1 : Scope
  Scope3 : Scope
  Sum1 : Sum  Inputs=|-+  SaturateOnIntegerOverflow=on
  Sum3 : Sum  Inputs=|+-  SaturateOnIntegerOverflow=on
  Out1 : Outport
  Out2 : Outport  Port=2
  wires:
  Product3/1 -> Sum3/2
  Product4/1 -> Sum3/1
  2/1 -> Math Function2/1
  Math Function1/1 -> Product10/1, Product3/2
  a/1 -> Product4/2, Product3/3, Product10/3, Sum1/2
  ti/1 -> Math Function1/1
  Sum3/1 -> Out2/1, Scope1/1
  Math Function2/1 -> Product3/1
  t/1 -> Math Function3/1, Product10/2, Product4/1
  Math Function3/1 -> Product3/4
  Sum1/1 -> Out1/1, Scope3/1
  Product10/1 -> Sum1/1

== system model_min_mine/5 систем підйому/6/6-періодні/6-ти періодна криволінійна/пакет2 ==
  ti : Inport
  t : Inport  Port=2
  a : Inport  Port=3
  2 : Constant  Value=2
  Math Function1 : Math  Operator=reciprocal  SaturateOnIntegerOverflow=on
  Math Function2 : Math  Operator=reciprocal  SaturateOnIntegerOverflow=on
  Math Function3 : Math  Operator=square  SaturateOnIntegerOverflow=on
  Product10 : Product  Inputs=3  SaturateOnIntegerOverflow=on  OutDataTypeStr=Inherit: Same as first input
  Product3 : Product  Inputs=4  SaturateOnIntegerOverflow=on  OutDataTypeStr=Inherit: Same as first input
  Out1 : Outport
  Out2 : Outport  Port=2
  wires:
  2/1 -> Math Function2/1
  Product10/1 -> Out1/1
  Math Function1/1 -> Product10/1, Product3/2
  a/1 -> Product10/3, Product3/3
  ti/1 -> Math Function1/1
  Math Function2/1 -> Product3/1
  t/1 -> Math Function3/1, Product10/2
  Math Function3/1 -> Product3/4
  Product3/1 -> Out2/1

== system model_min_mine/5 систем підйому/6/6-періодні/6-ти періодна криволінійна/постійні ==
  Sum1 : Sum  Inputs=|++++++  SaturateOnIntegerOverflow=on
  Sum2 : Sum  Inputs=|+++  SaturateOnIntegerOverflow=on
  Sum3 : Sum  Inputs=|+++  SaturateOnIntegerOverflow=on
  a1 : Constant  Value=0.5
  a2 : Constant  Value=3
  "a4 " : Constant  Value=-3
  a5 : Constant  Value=-0.5
  t1 : Constant  Value=0.5
  t2 : Constant  Value=3.5
  t3 : Constant  Value=4
  t4 : Constant  Value=3.5
  "t4/ " : Constant  Value=0.5
  t5 : Constant  Value=0.5
  Out1 : Outport
  Out2 : Outport  Port=2
  Out3 : Outport  Port=3
  Out4 : Outport  Port=4
  Out5 : Outport  Port=5
  Out6 : Outport  Port=6
  Out7 : Outport  Port=7
  Out8 : Outport  Port=8
  Out9 : Outport  Port=9
  wires:
  a1/1 -> Out1/1
  "a4 "/1 -> Out3/1
  a5/1 -> Out4/1
  a2/1 -> Out2/1
  t1/1 -> Out5/1, Sum1/1, Sum2/1
  t3/1 -> Sum1/3, Sum2/3
  t2/1 -> Out6/1, Sum1/2, Sum2/2
  t5/1 -> Sum1/5
  t4/1 -> Out7/1, Sum1/4, Sum3/1
  Sum1/1 -> Out9/1
  Sum2/1 -> Sum3/2
  Sum3/1 -> Out8/1
  "t4/ "/1 -> Sum3/3, Sum1/6

== system model_min_mine/5 систем підйому/6/6-періодні/6-ти періодна пр/Subsystem ==
  t1 : Inport
  t : Inport  Port=2
  a1 : Inport  Port=3
  Constant5 : Constant
  Scope2 : Scope
  Sum4 : Sum  Inputs=|+-  SaturateOnIntegerOverflow=on
  Switch1 : Switch  Criteria=u2 ~= 0  RndMeth=Zero  SaturateOnIntegerOverflow=on
  Генераці : Subsystem  TreatAsAtomicUnit=on
  Out1 : Outport
  wires:
  Генераці/1(Out1) -> Switch1/2
  Sum4/1 -> Генераці/Trigger
  Constant5/1 -> Генераці/1(In1)
  t/1 -> Sum4/2
  t1/1 -> Sum4/1
  Switch1/1 -> Out1/1, Scope2/1
  a1/1 -> Switch1/3

== system model_min_mine/5 систем підйому/6/6-періодні/6-ти періодна пр/Subsystem1 ==
  t1 : Inport
  t : Inport  Port=2
  a1 : Inport  Port=3
  Constant5 : Constant
  Scope2 : Scope
  Sum4 : Sum  Inputs=|+-  SaturateOnIntegerOverflow=on
  Switch1 : Switch  Criteria=u2 ~= 0  RndMeth=Zero  SaturateOnIntegerOverflow=on
  Генераці : Subsystem  TreatAsAtomicUnit=on
  Out1 : Outport
  wires:
  Генераці/1(Out1) -> Switch1/2
  Sum4/1 -> Генераці/Trigger
  Constant5/1 -> Генераці/1(In1)
  t/1 -> Sum4/2
  t1/1 -> Sum4/1
  Switch1/1 -> Out1/1, Scope2/1
  a1/1 -> Switch1/3

== system model_min_mine/5 систем підйому/6/6-періодні/6-ти періодна пр/Subsystem2 ==
  t1 : Inport
  t : Inport  Port=2
  a1 : Inport  Port=3
  Constant5 : Constant
  Scope2 : Scope
  Scope8 : Scope
  Sum4 : Sum  Inputs=|+-  SaturateOnIntegerOverflow=on
  Switch1 : Switch  Criteria=u2 ~= 0  RndMeth=Zero  SaturateOnIntegerOverflow=on
  Генераці : Subsystem  TreatAsAtomicUnit=on
  Out1 : Outport
  wires:
  Генераці/1(Out1) -> Switch1/2
  Sum4/1 -> Генераці/Trigger
  Constant5/1 -> Генераці/1(In1)
  t/1 -> Sum4/2
  t1/1 -> Sum4/1
  Switch1/1 -> Scope2/1, Out1/1, Scope8/1
  a1/1 -> Switch1/1

== system model_min_mine/5 систем підйому/6/6-періодні/6-ти періодна пр/Subsystem3 ==
  t1 : Inport
  t : Inport  Port=2
  a1 : Inport  Port=3
  Constant5 : Constant
  Scope2 : Scope
  Sum4 : Sum  Inputs=|+-  SaturateOnIntegerOverflow=on
  Switch1 : Switch  Criteria=u2 ~= 0  RndMeth=Zero  SaturateOnIntegerOverflow=on
  Генераці : Subsystem  TreatAsAtomicUnit=on
  Out1 : Outport
  wires:
  Генераці/1(Out1) -> Switch1/2
  Sum4/1 -> Генераці/Trigger
  Constant5/1 -> Генераці/1(In1)
  t/1 -> Sum4/2
  t1/1 -> Sum4/1
  Switch1/1 -> Out1/1, Scope2/1
  a1/1 -> Switch1/1

== system model_min_mine/5 систем підйому/6/6-періодні/6-ти періодна пр/Subsystem6 ==
  Сума t : Inport
  t : Inport  Port=2
  a : Inport  Port=3
  Constant5 : Constant
  Sum4 : Sum  Inputs=|+-  SaturateOnIntegerOverflow=on
  Switch1 : Switch  Criteria=u2 ~= 0  RndMeth=Zero  SaturateOnIntegerOverflow=on
  Генераці : Subsystem  TreatAsAtomicUnit=on
  Out1 : Outport
  wires:
  Генераці/1(Out1) -> Switch1/2
  Sum4/1 -> Генераці/Trigger
  Constant5/1 -> Генераці/1(In1)
  t/1 -> Sum4/2
  Сума t/1 -> Sum4/1
  Switch1/1 -> Out1/1
  a/1 -> Switch1/3

== system model_min_mine/5 систем підйому/6/6-періодні/6-ти періодна пр/Допоміжний ==
  t1 : Inport
  t : Inport  Port=2
  a1 : Inport  Port=3
  Constant5 : Constant
  Scope2 : Scope
  Sum4 : Sum  Inputs=|+-  SaturateOnIntegerOverflow=on
  Switch1 : Switch  Criteria=u2 ~= 0  RndMeth=Zero  SaturateOnIntegerOverflow=on
  Генераці : Subsystem  TreatAsAtomicUnit=on
  Out1 : Outport
  wires:
  Генераці/1(Out1) -> Switch1/2
  Sum4/1 -> Генераці/Trigger
  Constant5/1 -> Генераці/1(In1)
  t/1 -> Sum4/2
  t1/1 -> Sum4/1
  Switch1/1 -> Out1/1, Scope2/1
  a1/1 -> Switch1/1

== system model_min_mine/5 систем підйому/6/6-періодні/6-ти періодна пр/Допоміжний1 ==
  t1 : Inport
  t : Inport  Port=2
  a1 : Inport  Port=3
  Constant5 : Constant
  Scope2 : Scope
  Sum4 : Sum  Inputs=|+-  SaturateOnIntegerOverflow=on
  Switch1 : Switch  Criteria=u2 ~= 0  RndMeth=Zero  SaturateOnIntegerOverflow=on
  Генераці : Subsystem  TreatAsAtomicUnit=on
  Out1 : Outport
  wires:
  Генераці/1(Out1) -> Switch1/2
  Sum4/1 -> Генераці/Trigger
  Constant5/1 -> Генераці/1(In1)
  t/1 -> Sum4/2
  t1/1 -> Sum4/1
  Switch1/1 -> Out1/1, Scope2/1
  a1/1 -> Switch1/3

== system model_min_mine/5 систем підйому/6/6-періодні/6-ти періодна пр/постійні ==
  Sum1 : Sum  Inputs=|++++++  SaturateOnIntegerOverflow=on
  Sum2 : Sum  Inputs=|+++  SaturateOnIntegerOverflow=on
  Sum3 : Sum  Inputs=|+++  SaturateOnIntegerOverflow=on
  a1 : Constant  Value=0.5
  a2 : Constant  Value=1.5
  "a4 " : Constant  Value=-1.5
  a5 : Constant  Value=-0.5
  t1 : Constant  Value=0.5
  t2 : Constant  Value=3.5
  t3 : Constant  Value=4
  t4 : Constant  Value=3.5
  "t4/ " : Constant  Value=0.5
  t5 : Constant  Value=0.5
  Out1 : Outport
  Out2 : Outport  Port=2
  Out3 : Outport  Port=3
  Out4 : Outport  Port=4
  Out5 : Outport  Port=5
  Out6 : Outport  Port=6
  Out7 : Outport  Port=7
  Out8 : Outport  Port=8
  Out9 : Outport  Port=9
  Out10 : Outport  Port=10
  wires:
  a1/1 -> Out1/1
  "a4 "/1 -> Out3/1
  a5/1 -> Out4/1
  a2/1 -> Out2/1
  t1/1 -> Out5/1, Sum1/1, Sum2/1
  t3/1 -> Sum1/3, Sum2/3
  t2/1 -> Out6/1, Sum1/2, Sum2/2
  t5/1 -> Sum1/5
  t4/1 -> Out7/1, Sum1/4, Sum3/1
  Sum1/1 -> Out9/1
  Sum2/1 -> Out10/1, Sum3/2
  Sum3/1 -> Out8/1
  "t4/ "/1 -> Sum3/3, Sum1/6

== system model_min_mine/5 систем підйому/6/7-періодні/7-ми періодна криволінійна/Subsystem ==
  t1 : Inport
  t : Inport  Port=2
  a1 : Inport  Port=3
  Constant5 : Constant
  Scope2 : Scope
  Sum4 : Sum  Inputs=|+-  SaturateOnIntegerOverflow=on
  Switch1 : Switch  Criteria=u2 ~= 0  RndMeth=Zero  SaturateOnIntegerOverflow=on
  Генераці : Subsystem  TreatAsAtomicUnit=on
  Out1 : Outport
  wires:
  Генераці/1(Out1) -> Switch1/2
  Sum4/1 -> Генераці/Trigger
  Constant5/1 -> Генераці/1(In1)
  t/1 -> Sum4/2
  t1/1 -> Sum4/1
  Switch1/1 -> Out1/1, Scope2/1
  a1/1 -> Switch1/3

== system model_min_mine/5 систем підйому/6/7-періодні/7-ми періодна криволінійна/Subsystem3 ==
  t1 : Inport
  t : Inport  Port=2
  a1 : Inport  Port=3
  Constant5 : Constant
  Scope2 : Scope
  Sum4 : Sum  Inputs=|+-  SaturateOnIntegerOverflow=on
  Switch1 : Switch  Criteria=u2 ~= 0  RndMeth=Zero  SaturateOnIntegerOverflow=on
  Генераці : Subsystem  TreatAsAtomicUnit=on
  Out1 : Outport
  wires:
  Генераці/1(Out1) -> Switch1/2
  Sum4/1 -> Генераці/Trigger
  Constant5/1 -> Генераці/1(In1)
  t/1 -> Sum4/2
  t1/1 -> Sum4/1
  Switch1/1 -> Out1/1, Scope2/1
  a1/1 -> Switch1/1

== system model_min_mine/5 систем підйому/6/7-періодні/7-ми періодна криволінійна/Subsystem6 ==
  Сума t : Inport
  t : Inport  Port=2
  a : Inport  Port=3
  Constant5 : Constant
  Sum4 : Sum  Inputs=|+-  SaturateOnIntegerOverflow=on
  Switch1 : Switch  Criteria=u2 ~= 0  RndMeth=Zero  SaturateOnIntegerOverflow=on
  Генераці : Subsystem  TreatAsAtomicUnit=on
  Out1 : Outport
  wires:
  Генераці/1(Out1) -> Switch1/2
  Sum4/1 -> Генераці/Trigger
  Constant5/1 -> Генераці/1(In1)
  t/1 -> Sum4/2
  Сума t/1 -> Sum4/1
  Switch1/1 -> Out1/1
  a/1 -> Switch1/3

== system model_min_mine/5 систем підйому/6/7-періодні/7-ми періодна криволінійна/Допоміжний ==
  t1 : Inport
  t : Inport  Port=2
  a1 : Inport  Port=3
  Constant5 : Constant
  Scope2 : Scope
  Sum4 : Sum  Inputs=|+-  SaturateOnIntegerOverflow=on
  Switch1 : Switch  Criteria=u2 ~= 0  RndMeth=Zero  SaturateOnIntegerOverflow=on
  Генераці : Subsystem  TreatAsAtomicUnit=on
  Out1 : Outport
  wires:
  Генераці/1(Out1) -> Switch1/2
  Sum4/1 -> Генераці/Trigger
  Constant5/1 -> Генераці/1(In1)
  t/1 -> Sum4/2
  t1/1 -> Sum4/1
  Switch1/1 -> Out1/1, Scope2/1
  a1/1 -> Switch1/1

== system model_min_mine/5 систем підйому/6/7-періодні/7-ми періодна криволінійна/Допоміжний1 ==
  t1 : Inport
  t : Inport  Port=2
  a1 : Inport  Port=3
  Constant5 : Constant
  Scope2 : Scope
  Sum4 : Sum  Inputs=|+-  SaturateOnIntegerOverflow=on
  Switch1 : Switch  Criteria=u2 ~= 0  RndMeth=Zero  SaturateOnIntegerOverflow=on
  Генераці : Subsystem  TreatAsAtomicUnit=on
  Out1 : Outport
  wires:
  Генераці/1(Out1) -> Switch1/2
  Sum4/1 -> Генераці/Trigger
  Constant5/1 -> Генераці/1(In1)
  t/1 -> Sum4/2
  t1/1 -> Sum4/1
  Switch1/1 -> Out1/1, Scope2/1
  a1/1 -> Switch1/3

== system model_min_mine/5 систем підйому/6/7-періодні/7-ми періодна криволінійна/пакет1 ==
  ti : Inport
  t : Inport  Port=2
  a : Inport  Port=3
  2 : Constant  Value=2
  Math Function1 : Math  Operator=reciprocal  SaturateOnIntegerOverflow=on
  Math Function2 : Math  Operator=reciprocal  SaturateOnIntegerOverflow=on
  Math Function3 : Math  Operator=square  SaturateOnIntegerOverflow=on
  Product10 : Product  Inputs=3  SaturateOnIntegerOverflow=on  OutDataTypeStr=Inherit: Same as first input
  Product3 : Product  Inputs=4  SaturateOnIntegerOverflow=on  OutDataTypeStr=Inherit: Same as first input
  Product4 : Product  SaturateOnIntegerOverflow=on  OutDataTypeStr=Inherit: Same as first input
  Scope1 : Scope
  Scope3 : Scope
  Sum1 : Sum  Inputs=|-+  SaturateOnIntegerOverflow=on
  Sum3 : Sum  Inputs=|+-  SaturateOnIntegerOverflow=on
  Out1 : Outport
  Out2 : Outport  Port=2
  wires:
  Product3/1 -> Sum3/2
  Product4/1 -> Sum3/1
  2/1 -> Math Function2/1
  Math Function1/1 -> Product10/1, Product3/2
  a/1 -> Product4/2, Product3/3, Product10/3, Sum1/2
  ti/1 -> Math Function1/1
  Sum3/1 -> Out2/1, Scope1/1
  Math Function2/1 -> Product3/1
  t/1 -> Math Function3/1, Product10/2, Product4/1
  Math Function3/1 -> Product3/4
  Sum1/1 -> Out1/1, Scope3/1
  Product10/1 -> Sum1/1

== system model_min_mine/5 систем підйому/6/7-періодні/7-ми періодна криволінійна/пакет2 ==
  ti : Inport
  t : Inport  Port=2
  a : Inport  Port=3
  2 : Constant  Value=2
  Math Function1 : Math  Operator=reciprocal  SaturateOnIntegerOverflow=on
  Math Function2 : Math  Operator=reciprocal  SaturateOnIntegerOverflow=on
  Math Function3 : Math  Operator=square  SaturateOnIntegerOverflow=on
  Product10 : Product  Inputs=3  SaturateOnIntegerOverflow=on  OutDataTypeStr=Inherit: Same as first input
  Product3 : Product  Inputs=4  SaturateOnIntegerOverflow=on  OutDataTypeStr=Inherit: Same as first input
  Out1 : Outport
  Out2 : Outport  Port=2
  wires:
  2/1 -> Math Function2/1
  Product10/1 -> Out1/1
  Math Function1/1 -> Product10/1, Product3/2
  a/1 -> Product10/3, Product3/3
  ti/1 -> Math Function1/1
  Math Function2/1 -> Product3/1
  t/1 -> Math Function3/1, Product10/2
  Math Function3/1 -> Product3/4
  Product3/1 -> Out2/1

== system model_min_mine/5 систем підйому/6/7-періодні/7-ми періодна криволінійна/постійні ==
  Sum1 : Sum  Inputs=|+++++++  SaturateOnIntegerOverflow=on
  Sum2 : Sum  Inputs=|+++  SaturateOnIntegerOverflow=on
  Sum3 : Sum  Inputs=|+++  SaturateOnIntegerOverflow=on
  Sum4 : Sum  Inputs=|++  SaturateOnIntegerOverflow=on
  a1 : Constant  Value=0.5
  a2 : Constant  Value=1.5
  "a4 " : Constant  Value=-1.5
  a5 : Constant  Value=-0.5
  t1 : Constant  Value=0.5
  "t1/ " : Constant  Value=0.5
  t2 : Constant  Value=3.5
  t3 : Constant  Value=4
  t4 : Constant  Value=3.5
  "t4/ " : Constant  Value=0.5
  t5 : Constant  Value=0.5
  Out1 : Outport
  Out2 : Outport  Port=2
  Out3 : Outport  Port=3
  Out4 : Outport  Port=4
  Out5 : Outport  Port=5
  Out6 : Outport  Port=6
  Out7 : Outport  Port=7
  Out8 : Outport  Port=8
  Out9 : Outport  Port=9
  Out10 : Outport  Port=10
  Out11 : Outport  Port=11
  wires:
  a1/1 -> Out1/1
  "a4 "/1 -> Out3/1
  a5/1 -> Out4/1
  a2/1 -> Out2/1
  t1/1 -> Out5/1, Sum1/1, Sum2/1, Sum4/1
  t3/1 -> Sum1/3, Sum2/3
  t2/1 -> Out6/1, Sum1/2, Sum2/2
  t5/1 -> Sum1/5
  t4/1 -> Out7/1, Sum1/4, Sum3/1
  Sum1/1 -> Out9/1
  Sum2/1 -> Out10/1, Sum3/2
  Sum3/1 -> Out8/1
  "t4/ "/1 -> Sum3/3, Sum1/6
  "t1/ "/1 -> Sum1/7, Sum4/2
  Sum4/1 -> Out11/1

== system model_min_mine/5 систем підйому/6/7-періодні/7-ми періодна пр/Subsystem ==
  t1 : Inport
  t : Inport  Port=2
  a1 : Inport  Port=3
  Constant5 : Constant
  Scope2 : Scope
  Sum4 : Sum  Inputs=|+-  SaturateOnIntegerOverflow=on
  Switch1 : Switch  Criteria=u2 ~= 0  RndMeth=Zero  SaturateOnIntegerOverflow=on
  Генераці : Subsystem  TreatAsAtomicUnit=on
  Out1 : Outport
  wires:
  Генераці/1(Out1) -> Switch1/2
  Sum4/1 -> Генераці/Trigger
  Constant5/1 -> Генераці/1(In1)
  t/1 -> Sum4/2
  t1/1 -> Sum4/1
  Switch1/1 -> Out1/1, Scope2/1
  a1/1 -> Switch1/3

== system model_min_mine/5 систем підйому/6/7-періодні/7-ми періодна пр/Subsystem1 ==
  t1 : Inport
  t : Inport  Port=2
  a1 : Inport  Port=3
  Constant5 : Constant
  Scope2 : Scope
  Sum4 : Sum  Inputs=|+-  SaturateOnIntegerOverflow=on
  Switch1 : Switch  Criteria=u2 ~= 0  RndMeth=Zero  SaturateOnIntegerOverflow=on
  Генераці : Subsystem  TreatAsAtomicUnit=on
  Out1 : Outport
  wires:
  Генераці/1(Out1) -> Switch1/2
  Sum4/1 -> Генераці/Trigger
  Constant5/1 -> Генераці/1(In1)
  t/1 -> Sum4/2
  t1/1 -> Sum4/1
  Switch1/1 -> Out1/1, Scope2/1
  a1/1 -> Switch1/3

== system model_min_mine/5 систем підйому/6/7-періодні/7-ми періодна пр/Subsystem2 ==
  t1 : Inport
  t : Inport  Port=2
  a1 : Inport  Port=3
  Constant5 : Constant
  Scope2 : Scope
  Scope8 : Scope
  Sum4 : Sum  Inputs=|+-  SaturateOnIntegerOverflow=on
  Switch1 : Switch  Criteria=u2 ~= 0  RndMeth=Zero  SaturateOnIntegerOverflow=on
  Генераці : Subsystem  TreatAsAtomicUnit=on
  Out1 : Outport
  wires:
  Генераці/1(Out1) -> Switch1/2
  Sum4/1 -> Генераці/Trigger
  Constant5/1 -> Генераці/1(In1)
  t/1 -> Sum4/2
  t1/1 -> Sum4/1
  Switch1/1 -> Scope2/1, Out1/1, Scope8/1
  a1/1 -> Switch1/1
